simulink model "dyskretne_simulink"  (R2022b)
settings: Solver=ode4  StartTime=0.0  StopTime=20  FixedStep=0.001  RelTol=1e-3
undefined symbols (not defined in the file): A, A_plus, B, B_plus, C, C_plus, D, D_plus, h
settings Model: Creator=Andrzej  LastModifiedBy=Andrzej

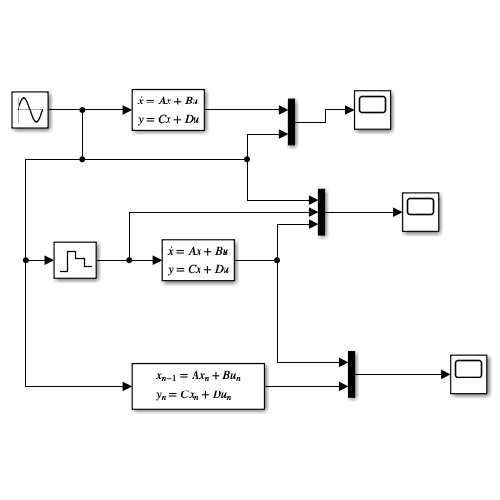
[thumbnail: Simulink's stored preview of the top-level diagram]
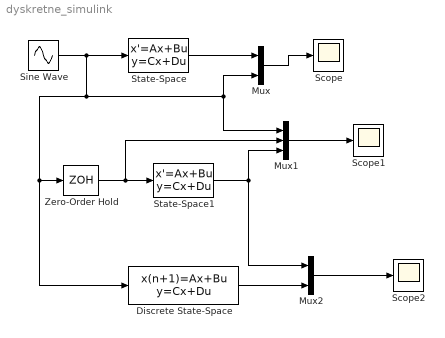
== system dyskretne_simulink ==
  Discrete State-Space : DiscreteStateSpace  A=A_plus  B=B_plus  C=C_plus  D=D_plus  InitialCondition=[1;0]  SampleTime=round(h,3)
  Mux : Mux  Inputs=2
  Mux1 : Mux  Inputs=3
  Mux2 : Mux  Inputs=2
  Scope : Scope
  Scope1 : Scope
  Scope2 : Scope
  Sine Wave : Sin  Bias=1  SampleTime=0
  State-Space : StateSpace  A=A  B=B  C=C  D=D  InitialCondition=[1; 0]
  State-Space1 : StateSpace  A=A  B=B  C=C  D=D  InitialCondition=[1;0]
  Zero-Order Hold : ZeroOrderHold  SampleTime=round(h, 3)
  wires:
  Sine Wave/1 -> Discrete State-Space/1, Zero-Order Hold/1, Mux1/1, Mux/2, State-Space/1
  State-Space/1 -> Mux/1
  Mux/1 -> Scope/1
  Zero-Order Hold/1 -> Mux1/2, State-Space1/1
  Mux1/1 -> Scope1/1
  State-Space1/1 -> Mux2/1, Mux1/3
  Mux2/1 -> Scope2/1
  Discrete State-Space/1 -> Mux2/2
